simulink model "downsample_ref2"  (Simulink 4.00)
settings: Solver=FixedStepDiscrete  StartTime=0.0  StopTime=5  RelTol=1e-3
PreLoadFcn:
  | load mtlb, whos mtlb Fs
PostLoadFcn:
  | set_param(gcs,'SimulationCommand','Update')
libraries: dspsigops x1, dspsrcs3 x1
settings Model: RequirementInfo=9  LastModifiedBy=dfass  LimitDataPoints=off  ExtModeTrigMode=oneshot  ExtModeArmWhenConnect=off  BlockReductionOpt=off

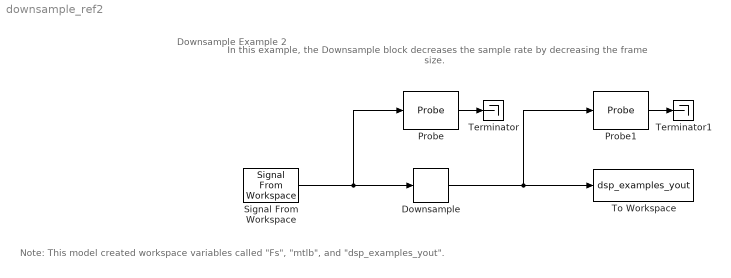
== system downsample_ref2 ==
  note: Downsample Example 2
  note: In this example, the Downsample block decreases
      | the sample rate by decreasing the frame size.
  note: Note: This model created workspace variables called "Fs", "mtlb", and "dsp_examples_yout".
  Downsample : dspsigops/Downsample  N=4  phase=0  ic=0  smode=Allow multirate  fmode=Maintain input frame rate
  Probe : Probe  ProbeWidth=off  ProbeSampleTime=on  ProbeComplexSignal=off  ProbeSignalDimensions=off
  Probe1 : Probe  ProbeWidth=off  ProbeSampleTime=on  ProbeComplexSignal=off  ProbeSignalDimensions=off
  Signal From Workspace : dspsrcs3/Signal From Workspace  X=mtlb  Ts=1/64  nsamps=64  OutputAfterFinalValue=Setting To Zero
  Terminator : Terminator
  Terminator1 : Terminator
  To Workspace : ToWorkspace  VariableName=dsp_examples_yout  SampleTime=-1  SaveFormat=Array
  wires:
  Downsample/1 -> To Workspace/1, Probe1/1
  Signal From Workspace/1 -> Probe/1, Downsample/1
  Probe/1 -> Terminator/1
  Probe1/1 -> Terminator1/1
